simulink model "initial_condition"  (R2020b)
settings: Solver=VariableStepAuto  StartTime=0.0  StopTime=10.0  RelTol=1e-3
libraries: simulink x6
settings Model: Creator=Luke  LastModifiedBy=Luke

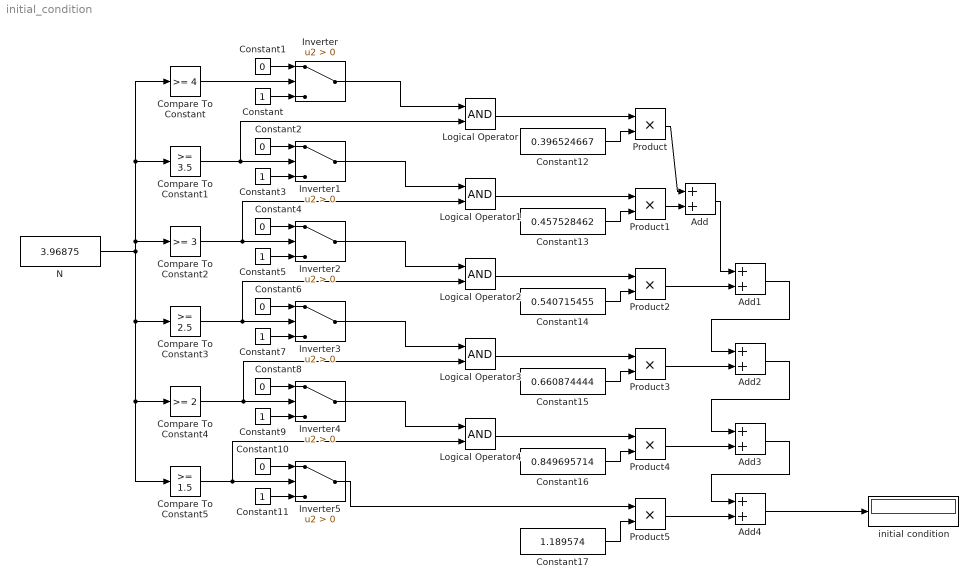
== system initial_condition ==
  Add{,1..4} (5 alike) : Sum
  Compare To Constant : simulink/Logic and Bit Operations/Compare To Constant  relop=>=  const=4  OutDataTypeStr=boolean
  Compare To Constant1 : simulink/Logic and Bit Operations/Compare To Constant  relop=>=  const=3.5  OutDataTypeStr=boolean
  Compare To Constant2 : simulink/Logic and Bit Operations/Compare To Constant  relop=>=  const=3  OutDataTypeStr=boolean
  Compare To Constant3 : simulink/Logic and Bit Operations/Compare To Constant  relop=>=  const=2.5  OutDataTypeStr=boolean
  Compare To Constant4 : simulink/Logic and Bit Operations/Compare To Constant  relop=>=  const=2  OutDataTypeStr=boolean
  Compare To Constant5 : simulink/Logic and Bit Operations/Compare To Constant  relop=>=  const=1.5  OutDataTypeStr=boolean
  Constant{,3,5,7,9,11} (6 alike) : Constant
  Constant{1..2,4,6,8,10} (6 alike) : Constant  Value=0
  Constant12 : Constant  Value=0.396524667
  Constant13 : Constant  Value=0.457528462
  Constant14 : Constant  Value=0.540715455
  Constant15 : Constant  Value=0.660874444
  Constant16 : Constant  Value=0.849695714
  Constant17 : Constant  Value=1.189574
  Inverter{,1..5} (6 alike) : Switch  Criteria=u2 > Threshold
  Logical Operator{,1..4} (5 alike) : Logic  AllPortsSameDT=off  OutDataTypeStr=boolean
  N : Constant  Value=3.96875
  Product{,1..5} (6 alike) : Product
  initial condition : Display
  wires:
  N/1 -> Compare To Constant5/1, Compare To Constant4/1, Compare To Constant3/1, Compare To Constant1/1, Compare To Constant/1, Compare To Constant2/1
  Compare To Constant/1 -> Inverter/2
  Constant/1 -> Inverter/3
  Constant1/1 -> Inverter/1
  Compare To Constant2/1 -> Inverter2/2, Logical Operator1/2
  Compare To Constant3/1 -> Inverter3/2, Logical Operator2/2
  Compare To Constant4/1 -> Logical Operator3/2, Inverter4/2
  Compare To Constant5/1 -> Logical Operator4/2, Inverter5/2
  Inverter/1 -> Logical Operator/1
  Compare To Constant1/1 -> Logical Operator/2, Inverter1/2
  Inverter1/1 -> Logical Operator1/1
  Inverter2/1 -> Logical Operator2/1
  Inverter3/1 -> Logical Operator3/1
  Inverter4/1 -> Logical Operator4/1
  Constant3/1 -> Inverter1/3
  Constant2/1 -> Inverter1/1
  Constant4/1 -> Inverter2/1
  Constant5/1 -> Inverter2/3
  Constant6/1 -> Inverter3/1
  Constant7/1 -> Inverter3/3
  Constant8/1 -> Inverter4/1
  Constant9/1 -> Inverter4/3
  Constant10/1 -> Inverter5/1
  Constant11/1 -> Inverter5/3
  Logical Operator/1 -> Product/1
  Constant12/1 -> Product/2
  Constant13/1 -> Product1/2
  Logical Operator1/1 -> Product1/1
  Constant14/1 -> Product2/2
  Logical Operator2/1 -> Product2/1
  Constant15/1 -> Product3/2
  Logical Operator3/1 -> Product3/1
  Constant16/1 -> Product4/2
  Logical Operator4/1 -> Product4/1
  Constant17/1 -> Product5/2
  Inverter5/1 -> Product5/1
  Product/1 -> Add/1
  Product1/1 -> Add/2
  Add/1 -> Add1/1
  Product2/1 -> Add1/2
  Add1/1 -> Add2/1
  Product3/1 -> Add2/2
  Add2/1 -> Add3/1
  Product4/1 -> Add3/2
  Add3/1 -> Add4/1
  Product5/1 -> Add4/2
  Add4/1 -> initial condition/1
